simulink model "EVPowertrain"  (R2018a)
settings: Solver=VariableStepAuto  StartTime=0  StopTime=200  RelTol=1e-3
libraries: fl_lib x7, nesl_utility x7, sdl_lib x6, elec_lib x4, autolibshared x2
settings Model: Creator=raiya  LastModifiedBy=raiya
settings SolverCC: ZeroCrossAlgorithm=Adaptive
settings DebuggingCC: MaxConsecutiveZCsMsg=none

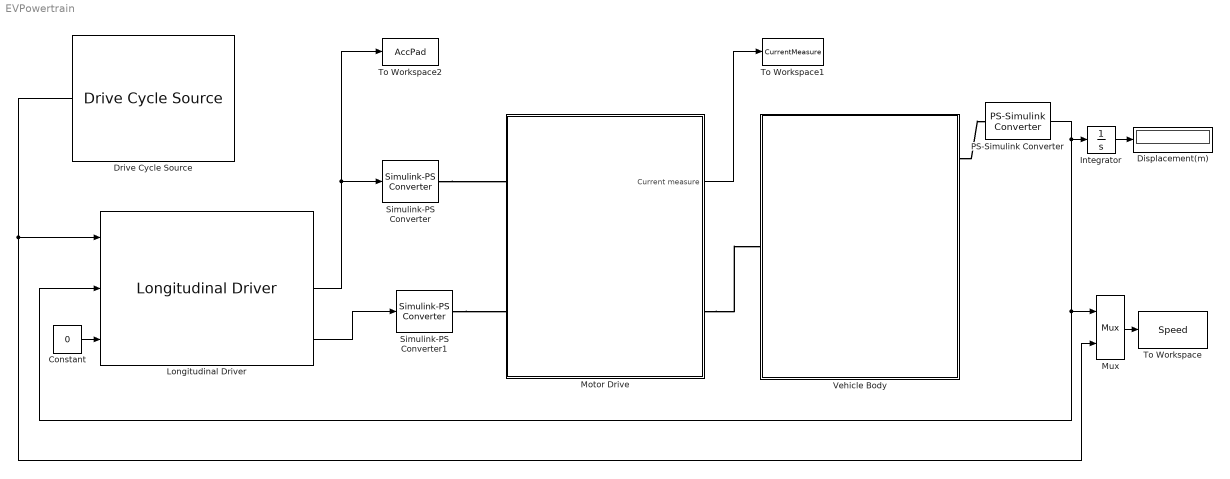
== system EVPowertrain ==
  Constant : Constant  Value=0
  "Displacement(m) " : Display
  Drive Cycle Source : autolibshared/Drive Cycle Source  cycleVar=ECE R15 (single cycle)  fileVar=cycleFTP75.mat  tfinal="195  seconds, Cyclic"  cycleRepeat=on  outAccPort=off  outGearPort=off  gearList=No gear data  t_wot1=5  xdot_woto=0  xdot_wot1=30  t_wot2=20  xdot_wot2=0  t_wotend=30  srcUnit=m/s  outUnit=m/s  srcAccUnit=m/s/s  outAccUnit=m/s^2  dt=0  aMode=1
      settings: SourceProductName=Powertrain Blockset  SourceProductBaseCode=PW
  Integrator : Integrator  InitialCondition=1
  Longitudinal Driver : autolibshared/Longitudinal Driver  aMode=2  vnom=5  Kp=10  Ki=5  Kaw=1  Kff=.1  Kg=0  tauerr=.01
      settings: SourceProductName=Powertrain Blockset  SourceProductBaseCode=PW
  Motor Drive : Subsystem
  Mux : Mux  Inputs=2
  PS-Simulink Converter : nesl_utility/PS-Simulink Converter  PhysicalDomain=network_engine_domain  SubClassName=ps_output  LeftPortType=input  RightPortType=output  PseudoPeriodic=off  Frequencies=[]  Unit=m/s  AffineConversion=off
  Simulink-PS Converter : nesl_utility/Simulink-PS Converter  PhysicalDomain=network_engine_domain  SubClassName=ps_input  LeftPortType=input  RightPortType=output  PseudoPeriodic=off  Frequencies=[]  NoiseDistribution=none  NoiseParameters=[]  Unit=1  AffineConversion=off  FilteringAndDerivatives=provide  SimscapeFilterOrder=1  InputFilterTimeConstant=0.001  UdotUserProvided=0
  Simulink-PS Converter1 : nesl_utility/Simulink-PS Converter  PhysicalDomain=network_engine_domain  SubClassName=ps_input  LeftPortType=input  RightPortType=output  PseudoPeriodic=off  Frequencies=[]  NoiseDistribution=none  NoiseParameters=[]  Unit=1  AffineConversion=off  FilteringAndDerivatives=provide  SimscapeFilterOrder=1  InputFilterTimeConstant=0.001  UdotUserProvided=0
  To Workspace : ToWorkspace  VariableName=Speed  SaveFormat=Timeseries  SampleTime=-1
  To Workspace1 : ToWorkspace  VariableName=CurrentMeasure  SaveFormat=Timeseries  SampleTime=-1
  To Workspace2 : ToWorkspace  VariableName=AccPad  SaveFormat=Timeseries  SampleTime=-1
  "Vehicle Body " : Subsystem
  wires:
  Drive Cycle Source/1 -> Longitudinal Driver/1, Mux/2
  Longitudinal Driver/2 -> Simulink-PS Converter/1, To Workspace2/1
  Longitudinal Driver/3 -> Simulink-PS Converter1/1
  PS-Simulink Converter/1 -> Integrator/1, Mux/1, Longitudinal Driver/2
  Constant/1 -> Longitudinal Driver/3
  Integrator/1 -> "Displacement(m) "/1
  Mux/1 -> To Workspace/1
  Motor Drive/1("Current measure ") -> To Workspace1/1
  connections:
  "Vehicle Body "/RConn1 -- PS-Simulink Converter/LConn1
  Motor Drive/RConn1 -- "Vehicle Body "/LConn2
  Simulink-PS Converter/RConn1 -- Motor Drive/LConn1
  Simulink-PS Converter1/RConn1 -- Motor Drive/LConn2

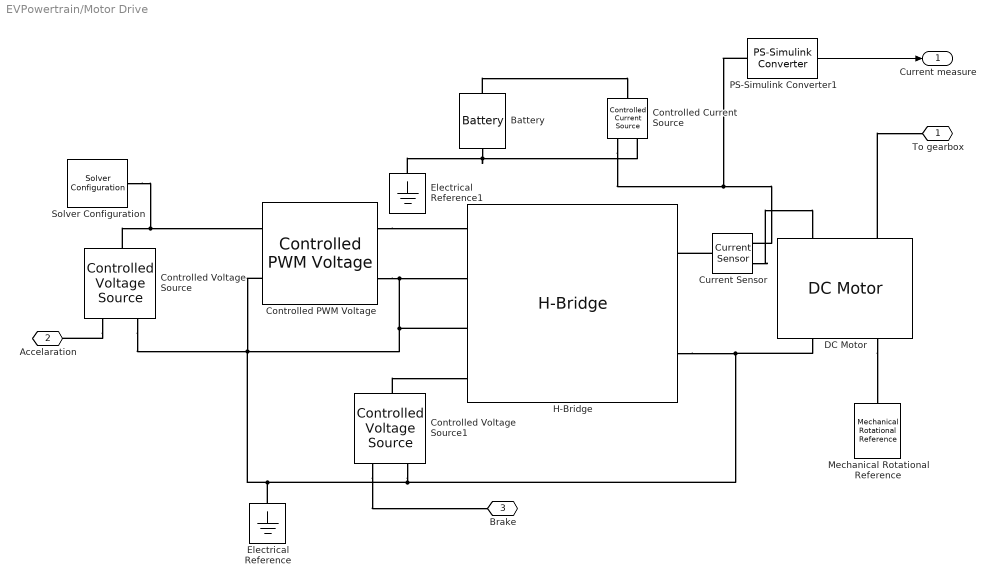
== system EVPowertrain/Motor Drive ==
  Battery : elec_lib/Sources/Battery  Vnom=500 V  R1=2 Ohm  prm_AH=1  AH=50 hr*A  V1=11.5 V  AH1=25 hr*A  prm_R2=1  R2=2000 Ohm  prm_dyn=1  Rp1=0.005 Ohm  tau1=30 s  Rp2=0.005 Ohm  tau2=30 s  prm_fade=1  N_fade=100  AH_fade=45 hr*A  R1_fade=2.02 Ohm  V1_fade=10.35 V  i_specify=off  i_priority=None  i=0 A  i_nominal_specify=off  i_nominal_unit=A  i_nominal_value=1  v_specify=off  v_priority=None  v=0 V  v_nominal_specify=off  v_nominal_unit=V  v_nominal_value=1  charge_specify=off  charge_priority=High  charge=50 hr*A  charge_nominal_specify=off  charge_nominal_unit=hr*A  charge_nominal_value=1  num_cycles_specify=off  num_cycles_priority=High  num_cycles=0  num_cycles_nominal_specify=off  num_cycles_nominal_unit=1  num_cycles_nominal_value=1  thermal_mass=30000 J/K  Tmeas=298.15 K  Vnom_T2=12 V  R1_T2=2.2 Ohm  V1_T2=11.4 V  R2_T2=2200 Ohm  Rp1_T2=0.005 Ohm  tau1_T2=30 s  Rp2_T2=0.005 Ohm  tau2_T2=30 s  Tmeas2=273.15 K  temperature_specify=off  temperature_priority=High  temperature=298.15 K  temperature_nominal_specify=off  temperature_nominal_unit=K  temperature_nominal_value=1
      settings: SourceProductName=Simscape Electronics  SourceProductBaseCode=SN
  Controlled Current Source : fl_lib/Electrical/Electrical Sources/Controlled Current Source
  Controlled PWM Voltage : elec_lib/Actuators & Drivers/Drivers/Controlled PWM Voltage  F=10 GHz  TD=0 s  pulse_width_offset=0 s  pulse_min=0 s  Vmin=0 V  Vmax=5 V  Vm=5 V  pwm_or_av=2  event_type=1  sample_time=1e-6 s  u_min=0  u_max=1
      settings: SourceProductName=Simscape Electronics  SourceProductBaseCode=SN
  Controlled Voltage Source : fl_lib/Electrical/Electrical Sources/Controlled Voltage Source
  Controlled Voltage Source1 : fl_lib/Electrical/Electrical Sources/Controlled Voltage Source
  Current Sensor : fl_lib/Electrical/Electrical Sensors/Current Sensor
  DC Motor : elec_lib/Actuators & Drivers/Rotational Actuators/DC Motor  parameterization=3  Ra=3.9 Ohm  La=12e-6 H  emf_or_torque=1  Kv=0.072e-3 V/rpm  Ki=6.876e-4 N*m/A  T_stall=0.24e-3 N*m  w_max=10000 rpm  w_rated=8000 rpm  P_rated=100 kW  V_rated=500 V  J=0.01 g*cm^2  lam_param=1  lam=.01 N*m/(rad/s)  i_noload=0 A  V_i_noload=1.5 V  speed0=0 rpm  alpha=3.93e-3 1/K  Tmeas=25 degC  thermal_mass=100 J/K  initial_temperature=25 degC
  Electrical Reference : fl_lib/Electrical/Electrical Elements/Electrical Reference
  Electrical Reference1 : fl_lib/Electrical/Electrical Elements/Electrical Reference
  H-Bridge : elec_lib/Actuators & Drivers/Drivers/H-Bridge  Venable=1 V  Vmax=5.0 V  Vreverse=1 V  Vbrake=1 V  Vm=500 V  pwm_or_av=2  discontinuous=0  freewheeling_mode=1  freewheeling_mode_disc=1  Ron=0.1 Ohm  Don=0.05 Ohm  Rload=10 Ohm  Lload=1e-5 H  F=10 kHz  thermal_mass=100 J/K  initial_temperature=298.15 K  Ron2=0.1 Ohm  Don2=0.05 Ohm  Tmeas=298.15 K  Tmeas2=398.15 K
      settings: SourceProductName=Simscape Electronics  SourceProductBaseCode=SN
  Mechanical Rotational Reference : fl_lib/Mechanical/Rotational Elements/Mechanical Rotational Reference
  PS-Simulink Converter1 : nesl_utility/PS-Simulink Converter  PhysicalDomain=network_engine_domain  SubClassName=ps_output  LeftPortType=input  RightPortType=output  PseudoPeriodic=off  Frequencies=[]  Unit=1  AffineConversion=off
  Solver Configuration : nesl_utility/Solver Configuration  PhysicalDomain=network_engine_domain  SubClassName=solver  LeftPortType=input  RightPortType=generic  Tones=[]  Harmonics=[]  SimulateNoise=off  Profile=off  UseLocalSampling=off  EnableSwitchedLinearOptims=on  FrequencyDomain=off  UseCCode=off  RelTol=0.001  AbsTol=1e-06  MinStep=1e-09  ToWorkspace=off  RevertToSquareIcSolve=off  NumHomotopyIterations=100  PhasorMode=off  PhasorModeNumHarmonics=1  DoDC=off  ResidualTolerance=1e-09  UseLocalSolver=off  LocalSolverChoice=NE_BACKWARD_EULER_ADVANCER  LocalSolverSampleTime=0.001  DoFixedCost=off  MaxNonlinIter=3  MaxModeIter=2  LinearAlgebra=Sparse  EquationFormulation=NE_TIME_EF  DelaysMemoryBudget=1024  AutomaticFiltering=on  FilteringTimeConstant=0.001
  "To gearbox " : PMIOPort  Side=Right
  Accelaration : PMIOPort  Port=2  Side=Left
  Brake : PMIOPort  Port=3  Side=Left
  "Current measure " : Outport
  wires:
  PS-Simulink Converter1/1 -> "Current measure "/1
  connections:
  Controlled Voltage Source/LConn1 -- Solver Configuration/RConn1 -- Controlled PWM Voltage/LConn1
  Controlled PWM Voltage/RConn1 -- H-Bridge/LConn1
  Battery/LConn1 -- Controlled Current Source/LConn1
  Controlled Current Source/RConn1 -- PS-Simulink Converter1/LConn1 -- Current Sensor/RConn1
  Controlled PWM Voltage/RConn2 -- Controlled PWM Voltage/LConn2 -- Controlled Voltage Source/RConn2 -- Controlled Voltage Source1/RConn2 -- DC Motor/RConn1 -- H-Bridge/RConn2 -- Electrical Reference/LConn1 -- H-Bridge/LConn3 -- H-Bridge/LConn2
  Current Sensor/LConn1 -- H-Bridge/RConn1
  Battery/RConn1 -- Electrical Reference1/LConn1 -- Controlled Current Source/RConn2
  Current Sensor/RConn2 -- DC Motor/LConn1
  DC Motor/RConn2 -- Mechanical Rotational Reference/LConn1
  Controlled Voltage Source1/LConn1 -- H-Bridge/LConn4
  DC Motor/LConn2 -- "To gearbox "/RConn1
  Controlled Voltage Source1/RConn1 -- Brake/RConn1
  Controlled Voltage Source/RConn1 -- Accelaration/RConn1

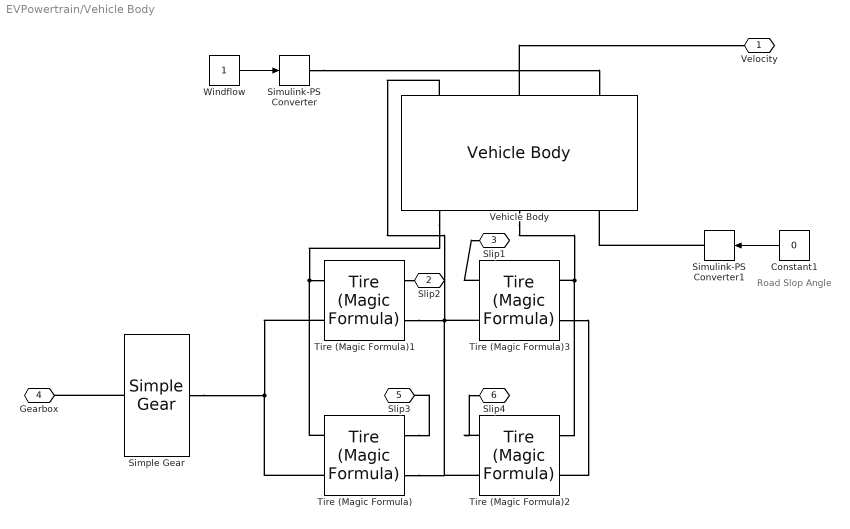
== system EVPowertrain/Vehicle Body  ==
  note: Road Slop Angle
  Constant1 : Constant  Value=0
  Simple Gear : sdl_lib/Gears/Simple Gear  ratio=3.7  rotation_direction=1  friction_model=1  T_noload=0.1 N*m  T_nom=5 N*m  efficiency_nom=0.8  efficiency=0.8  mu_visc=[0, 0] N*m/(rad/s)  w_thr=0.01 rad/s  pwr_thr=0.001 W  temperature_TLU=[280, 300, 320] K  load_TLU=[1, 5, 10] N*m  efficiency_TLU=[.95, .9, .85]  efficiency_TLU2=[.85, .8, .75; .95, .9, .85; .85, .8, .7]  thermal_mass=50 J/K  T_init=300 K
      settings: SourceProductName=Simscape Driveline
  Simulink-PS Converter : nesl_utility/Simulink-PS Converter  PhysicalDomain=network_engine_domain  SubClassName=ps_input  LeftPortType=input  RightPortType=output  PseudoPeriodic=off  Frequencies=[]  NoiseDistribution=none  NoiseParameters=[]  Unit=1  AffineConversion=off  FilteringAndDerivatives=provide  SimscapeFilterOrder=1  InputFilterTimeConstant=0.001  UdotUserProvided=0
  Simulink-PS Converter1 : nesl_utility/Simulink-PS Converter  PhysicalDomain=network_engine_domain  SubClassName=ps_input  LeftPortType=input  RightPortType=output  PseudoPeriodic=off  Frequencies=[]  NoiseDistribution=none  NoiseParameters=[]  Unit=1  AffineConversion=off  FilteringAndDerivatives=provide  SimscapeFilterOrder=1  InputFilterTimeConstant=0.001  UdotUserProvided=0
  Tire (Magic Formula) : sdl_lib/Tires & Vehicles/Tire (Magic Formula)  parameterization=1  F_z1=3000 N  F_x1=3500 N  kappa1=10  B_m=10  C_m=1.9  D_m=1  E_m=0.97  fz0=4000 N  p_Cx=1.685  p_Dx=[1.21, -.037]  p_Ex=[.344, .095, -.02, 0]  p_Kx=[21.51, -.163, .245]  p_Hx=[-.002, .002]  p_Vx=[0, 0]  v_tr_thr=0.1 m/s  r_e=0.3 m  model_compliance=0  stiffness=1e6 N/m  damping=1000 N/(m/s)  model_inertia=0  inertia=1 kg*m^2  initial_velocity=0 rad/s  model_resistance=0  resistance_model=1  coeff=0.015  p_tire=250e3 Pa  alpha=-0.003  beta=0.97  coeff_a=84e-4  coeff_b=6.2e-4 s/m  coeff_c=1.6e-4 s^2/m^2  v_thr=0.001 m/s
      settings: SourceProductName=Simscape Driveline
  Tire (Magic Formula)1 : sdl_lib/Tires & Vehicles/Tire (Magic Formula)  parameterization=2  F_z1=3000 N  F_x1=3500 N  kappa1=10  B_m=10  C_m=1.9  D_m=1  E_m=0.97  fz0=4000 N  p_Cx=1.685  p_Dx=[1.21, -.037]  p_Ex=[.344, .095, -.02, 0]  p_Kx=[21.51, -.163, .245]  p_Hx=[-.002, .002]  p_Vx=[0, 0]  v_tr_thr=0.1 m/s  r_e=0.3 m  model_compliance=0  stiffness=1e6 N/m  damping=1000 N/(m/s)  model_inertia=0  inertia=1 kg*m^2  initial_velocity=0 rad/s  model_resistance=1  resistance_model=1  coeff=0.015  p_tire=250e3 Pa  alpha=-0.003  beta=0.97  coeff_a=84e-4  coeff_b=6.2e-4 s/m  coeff_c=1.6e-4 s^2/m^2  v_thr=0.001 m/s
      settings: SourceProductName=Simscape Driveline
  Tire (Magic Formula)2 : sdl_lib/Tires & Vehicles/Tire (Magic Formula)  parameterization=1  F_z1=3000 N  F_x1=3500 N  kappa1=10  B_m=10  C_m=1.9  D_m=1  E_m=0.97  fz0=4000 N  p_Cx=1.685  p_Dx=[1.21, -.037]  p_Ex=[.344, .095, -.02, 0]  p_Kx=[21.51, -.163, .245]  p_Hx=[-.002, .002]  p_Vx=[0, 0]  v_tr_thr=0.1 m/s  r_e=0.3 m  model_compliance=0  stiffness=1e6 N/m  damping=1000 N/(m/s)  model_inertia=0  inertia=1 kg*m^2  initial_velocity=0 rad/s  model_resistance=0  resistance_model=1  coeff=0.015  p_tire=250e3 Pa  alpha=-0.003  beta=0.97  coeff_a=84e-4  coeff_b=6.2e-4 s/m  coeff_c=1.6e-4 s^2/m^2  v_thr=0.001 m/s
      settings: SourceProductName=Simscape Driveline
  Tire (Magic Formula)3 : sdl_lib/Tires & Vehicles/Tire (Magic Formula)  parameterization=1  F_z1=3000 N  F_x1=3500 N  kappa1=10  B_m=10  C_m=1.9  D_m=1  E_m=0.97  fz0=4000 N  p_Cx=1.685  p_Dx=[1.21, -.037]  p_Ex=[.344, .095, -.02, 0]  p_Kx=[21.51, -.163, .245]  p_Hx=[-.002, .002]  p_Vx=[0, 0]  v_tr_thr=0.1 m/s  r_e=0.3 m  model_compliance=0  stiffness=1e6 N/m  damping=1000 N/(m/s)  model_inertia=0  inertia=1 kg*m^2  initial_velocity=0 rad/s  model_resistance=0  resistance_model=1  coeff=0.015  p_tire=250e3 Pa  alpha=-0.003  beta=0.97  coeff_a=84e-4  coeff_b=6.2e-4 s/m  coeff_c=1.6e-4 s^2/m^2  v_thr=0.001 m/s
      settings: SourceProductName=Simscape Driveline
  Vehicle Body : sdl_lib/Tires & Vehicles/Vehicle Body  mass=400 kg  n_w=2  x_f=1.4 m  x_r=1.6 m  y_c=0.5 m  model_pitch=0  inertia=4000 kg*m^2  suspension_model=1  k_f=1e4 N/m  b_f=1e4 N/(m/s)  k_r=1e4 N/m  b_r=1e4 N/(m/s)  k_f_TLU=[-2000, -1000, 0, 1000, 2000] N  x_f_TLU=[-.4, -.2, 0, .2, .4] m  b_f_TLU=[-200, -100, 0, 100, 200] N  v_f_TLU=[-4, -2, 0, 2, 4] m/s  k_r_TLU=[-2000, -1000, 0, 1000, 2000] N  x_r_TLU=[-.4, -.2, 0, .2, .4] m  b_r_TLU=[-200, -100, 0, 100, 200] N  v_r_TLU=[-4, -2, 0, 2, 4] m/s  interp_method=simscape.enum.interpolation.linear  extrap_method=simscape.enum.extrapolation.linear  model_hardstop=0  upper_bound_f=.25 m  lower_bound_f=-.25 m  stop_k_f=1e6 N/m  stop_b_f=150 N/(m/s)  upper_bound_r=.25 m  lower_bound_r=-.25 m  stop_k_r=1e6 N/m  stop_b_r=150 N/(m/s)  initial_pitch=0 rad  initial_pitch_rate=0 rad/s  g=9.81 m/s^2  liftoff_warning=0  area=3 m^2  Cd=0.4  rho=1.18 kg/m^3  v_specify=off  v_priority=High  v=0 m/s  v_nominal_specify=off  v_nominal_unit=m/s  v_nominal_value=1
      settings: SourceProductName=Simscape Driveline
  "Windflow " : Constant
  Velocity : PMIOPort  Side=Right
  Slip2 : PMIOPort  Port=2  Side=Left
  Slip1 : PMIOPort  Port=3  Side=Right
  "Gearbox " : PMIOPort  Port=4  Side=Left
  Slip3 : PMIOPort  Port=5  Side=Left
  Slip4 : PMIOPort  Port=6  Side=Right
  wires:
  "Windflow "/1 -> Simulink-PS Converter/1
  Constant1/1 -> Simulink-PS Converter1/1
  connections:
  Tire (Magic Formula)2/RConn1 -- Slip4/RConn1
  Tire (Magic Formula)1/LConn2 -- Simple Gear/RConn1 -- Tire (Magic Formula)/LConn2
  Tire (Magic Formula)1/RConn2 -- Tire (Magic Formula)3/RConn2 -- Vehicle Body/LConn1 -- Tire (Magic Formula)/RConn2 -- Tire (Magic Formula)2/RConn2
  Tire (Magic Formula)3/LConn2 -- Tire (Magic Formula)2/LConn2
  Vehicle Body/RConn1 -- Tire (Magic Formula)/LConn1 -- Tire (Magic Formula)1/LConn1
  Vehicle Body/RConn2 -- Tire (Magic Formula)2/LConn1 -- Tire (Magic Formula)3/LConn1
  Tire (Magic Formula)3/RConn1 -- Slip1/RConn1
  Tire (Magic Formula)1/RConn1 -- Slip2/RConn1
  Simple Gear/LConn1 -- "Gearbox "/RConn1
  Tire (Magic Formula)/RConn1 -- Slip3/RConn1
  Vehicle Body/LConn2 -- Velocity/RConn1
  Simulink-PS Converter/RConn1 -- Vehicle Body/LConn3
  Simulink-PS Converter1/RConn1 -- Vehicle Body/RConn3
